simulink model "Ex4"  (R2013a)
settings: Solver=ode45  StartTime=0.0  StopTime=15  RelTol=1e-3
settings Model: Creator=Sudip Sinha  LastModifiedBy=Sudip Sinha

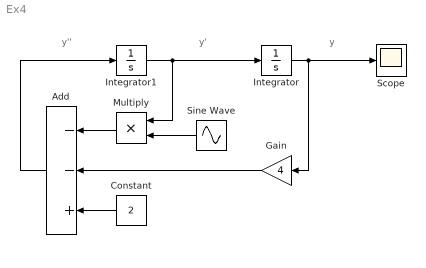
== system Ex4 ==
  note: y''
  note: y
  note: y'
  Add : Sum  Inputs=--+
  Constant : Constant  Value=2
  Gain : Gain  Gain=4
  Integrator : Integrator  InitialCondition=1
  Integrator1 : Integrator  InitialCondition=-1
  Multiply : Product  Inputs=**
  Scope : Scope
  Sine Wave : Sin  SampleTime=0
  wires:
  Integrator1/1 -> Multiply/1, Integrator/1
  Integrator/1 -> Scope/1, Gain/1
  Gain/1 -> Add/2
  Sine Wave/1 -> Multiply/2
  Multiply/1 -> Add/1
  Add/1 -> Integrator1/1
  Constant/1 -> Add/3
